simulink model "linearizationattempt"  (R2019b)
settings: Solver=ode15s  StartTime=0.0  StopTime=50  FixedStep=0.05  MaxStep=0.5  MinStep=0.01  RelTol=1e-1  AbsTol=1e-1
values from neighbouring files (symbols this model uses):
  x0 = [0, 0, 0.05, 2, 0, 0.01, 0.02, 0, 0, 0, 0, 0]    [createmodels.m]    (also in pidcontrolstartupscript.m = [0, 0, 0.05, 8, 0, 0.01, 0.02, 0, 0, 0, 0, 0])
undefined symbols (not defined in the file or in its folder): scalemodelstatefunction
libraries: aerolibanim x2, mpclib x1
settings Model: SimulationMode=accelerator  PacingRate=1000  Creator=Vlad  LastModifiedBy=Vlad
settings SolverCC: MaxConsecutiveMinStep=100
settings DataIOCC: ReturnWorkspaceOutputsName=tpe2155fcc_9c3f_42dd_9b90_435354f31060

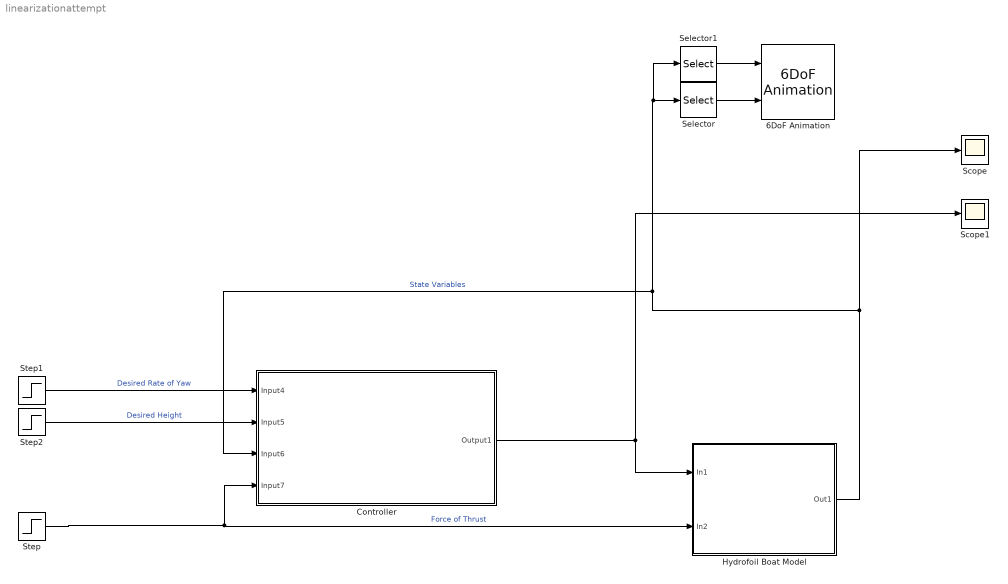
== system linearizationattempt ==
  6DoF Animation : aerolibanim/6DoF Animation  u1=[0 30 -2 2 -2 2]  u2=0.1  u3=1.0  u4=[4000 0 -5000]  u5=Fixed position  u6=[50 50 50]  u7=10  u8=on
      settings: SourceProductName=Aerospace Blockset
  Controller : Subsystem
  Hydrofoil Boat Model : Subsystem
  Scope : Scope
  Scope1 : Scope
  Selector : Selector  InputPortWidth=12  IndexOptions=Index vector (dialog)  Indices=[7 8 9]  OutputSizes=1
  Selector1 : Selector  InputPortWidth=12  IndexOptions=Index vector (dialog)  Indices=[1 2 3]  OutputSizes=1
  Step : Step  Time=0  After=100  SampleTime=0
  Step1 : Step  Time=0  After=0  SampleTime=0
  Step2 : Step  Time=0  After=0  SampleTime=0
  wires:
  Controller/1(Output1) -> Scope1/1, Hydrofoil Boat Model/1(In1)
  Hydrofoil Boat Model/1(Out1) -> Scope/1, Controller/3(Input6), Selector1/1, Selector/1  "State Variables"
  Step/1 -> Hydrofoil Boat Model/2(In2), Controller/4(Input7)  "Force of Thrust"
  Selector/1 -> 6DoF Animation/2
  Selector1/1 -> 6DoF Animation/1
  Step1/1 -> Controller/1(Input4)  "Desired Rate of Yaw"
  Step2/1 -> Controller/2(Input5)  "Desired Height"

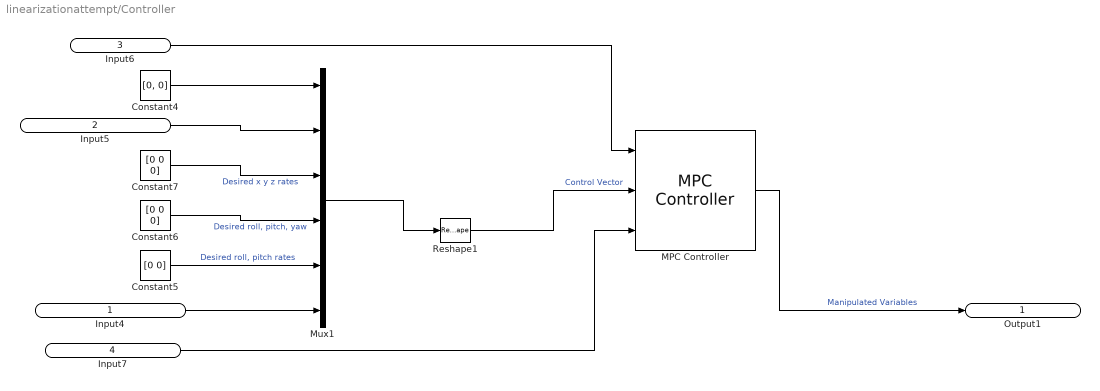
== system linearizationattempt/Controller ==
  Input4 : Inport
  Input5 : Inport  Port=2
  Input6 : Inport  Port=3
  Input7 : Inport  Port=4
  Constant4 : Constant  Value=[0, 0]
  Constant5 : Constant  Value=[0 0]
  Constant6 : Constant  Value=[0 0 0]
  Constant7 : Constant  Value=[0 0 0]
  MPC Controller : mpclib/MPC Controller  SCDEnableBlockLinearizationSpecification=on  mpcobj=mpc1  is_multiple=0  enable_value=0  return_u0=off  updateMPCinCallerWorkspace=on  md_inport=on  mv_inport=off  uref_inport=off  return_cost=off  return_mvseq=off  return_qpstatus=off  return_xseq=off  return_state=off  return_ovseq=off  state_inport=off  umin_inport=off  umax_inport=off  ymin_inport=off  ymax_inport=off  cc_inport=off  ywt_inport=off  uwt_inport=off  duwt_inport=off  rhoeps_inport=off  pm_inport=off  MaximumP=10  HorizonChoice=FixedHorizon  n_ts=0.1  n_p=10  n_mv=4  n_md=1  n_ud=0  n_mo=12  n_uo=0  BlockDataType=double  SampleTimeInherited=off  switch_inport=off
  Mux1 : Mux  Inputs=6
  Reshape1 : Reshape  OutputDimensionality=Row vector (2-D)
  Output1 : Outport
  wires:
  Constant5/1 -> Mux1/5  "Desired roll, pitch rates"
  Input4/1 -> Mux1/6
  Input7/1 -> MPC Controller/3
  Constant6/1 -> Mux1/4  "Desired roll, pitch, yaw"
  Constant4/1 -> Mux1/1
  Input5/1 -> Mux1/2
  Constant7/1 -> Mux1/3  "Desired x y z rates"
  Input6/1 -> MPC Controller/1
  Mux1/1 -> Reshape1/1
  Reshape1/1 -> MPC Controller/2  "Control Vector"
  MPC Controller/1 -> Output1/1  "Manipulated Variables"

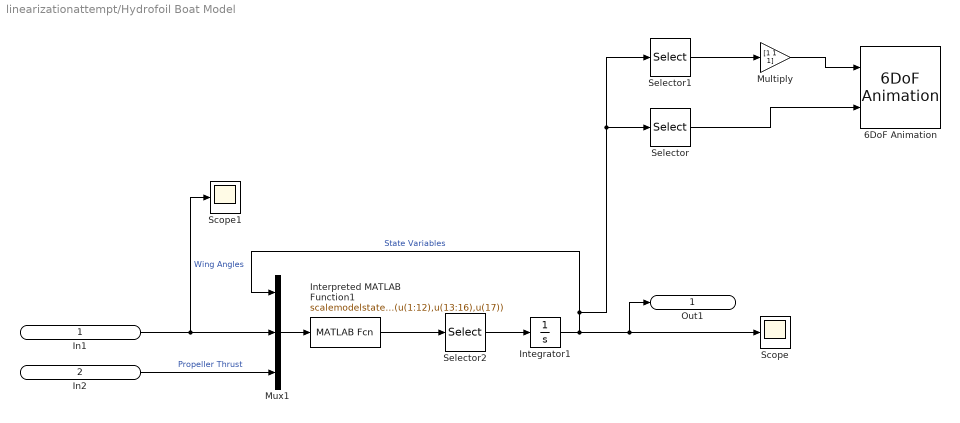
== system linearizationattempt/Hydrofoil Boat Model ==
  In1 : Inport
  In2 : Inport  Port=2
  6DoF Animation : aerolibanim/6DoF Animation  u1=[0 30 -2 2 -1 0]  u2=0.1  u3=5  u4=[4000 0 -5000]  u5=Fixed position  u6=[20 20 -20]  u7=20  u8=on
      settings: SourceProductName=Aerospace Blockset
  Integrator1 : Integrator  InitialCondition=x0
  Interpreted MATLAB Function1 : MATLABFcn  MATLABFcn=scalemodelstatefunction(u(1:12),u(13:16),u(17))  OutputDimensions=12
  Multiply : Gain  Gain=[1 1 1]
  Mux1 : Mux  Inputs=3
  Scope : Scope
  Scope1 : Scope
  Selector : Selector  InputPortWidth=12  IndexOptions=Index vector (dialog)  Indices=[8 7 9]  OutputSizes=1
  Selector1 : Selector  InputPortWidth=12  IndexOptions=Index vector (dialog)  Indices=[1 2 3]  OutputSizes=1
  Selector2 : Selector  InputPortWidth=12  IndexOptions=Index vector (dialog)  Indices=[1 2 3 4 5 6 7 8 9 10 11 12]  OutputSizes=1
  Out1 : Outport
  wires:
  In1/1 -> Scope1/1, Mux1/2  "Wing Angles"
  Interpreted MATLAB Function1/1 -> Selector2/1
  Mux1/1 -> Interpreted MATLAB Function1/1
  In2/1 -> Mux1/3  "Propeller Thrust"
  Selector1/1 -> Multiply/1
  Integrator1/1 -> Out1/1, Scope/1, Selector/1, Selector1/1, Mux1/1  "State Variables"
  Selector/1 -> 6DoF Animation/2
  Selector2/1 -> Integrator1/1
  Multiply/1 -> 6DoF Animation/1
